simulink library "follow_the_leader_library"  (R2018b)
settings: Solver=VariableStepAuto  StartTime=0.0  StopTime=10.0  RelTol=1e-3
undefined symbols (not defined in the file or in its folder): water, wr
settings Model: Creator=martin  LastModifiedBy=martin

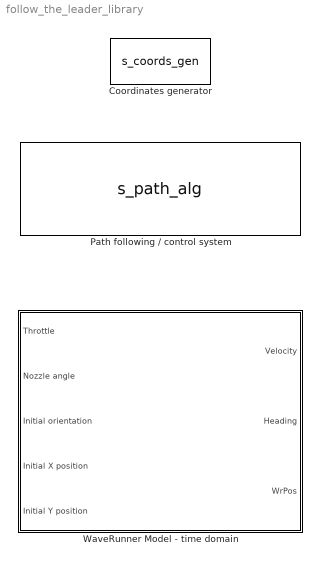
== system follow_the_leader_library ==
  Coordinates generator : S-Function  FunctionName=s_coords_gen  Parameters=steptime fname  SFunctionDeploymentMode=off  EnableBusSupport=off  mask(Coordinates generator){fname=../test1.txt, steptime=1}
      mask prompts: fname "File name"; steptime "Step time [coordinate / sec]"
      mask help:
      | Function simulating a GPS.
      |
      | The file must contain space separated GPS coordinates only, one coordinate / row.
      |
      | The step time controls the rate at which the coordinates are emitted.
      mask Display: fprintf('Coordinates\ngenerator')
  Path following / control system : S-Function  FunctionName=s_path_alg  Parameters=dt g_Kp g_Tf g_Kd g_Ki g_max g_min n_Kp n_Tf n_Kd n_Ki n_max n_min  SFunctionModules='path_alg'  SFunctionDeploymentMode=off  EnableBusSupport=off  mask(Path following / control system){dt=0.5, g_Kp=1.0, g_Tf=1.0, g_Kd=0.0, g_Ki=0.0, g_max=100, g_min=0, n_Kp=-1.0, n_Tf=1.0, n_Kd=0.0, n_Ki=0.0, n_max=6 * pi / 180, n_min=-6 * pi / 180}
      mask prompts: dt "Δt"; g_Kp "Kp"; g_Tf "Tf"; g_Kd "Kd"; g_Ki "Ki"; g_max "Max"; g_min "Min"; n_Kp "Kp"; n_Tf "Tf"; n_Kd "Kd"; n_Ki "Ki"; n_max "Max"; n_min "Min"
      mask DialogControl Container3 Prompt: Controller parameters - Gas
      mask DialogControl Container5 Prompt: Controller parameters - Nozzle angle
      mask Display:
      | text(0.5, 0.5, 'Path Following Algorithm /\nControl system', 'horizontalAlignment', 'center', 'verticalAlignment', 'middle')
      | port_label('input', 1, 'LC coordinates')
      | port_label('input', 2, 'WR position')
      | port_label('input', 3, 'WR angle')
      | port_label('input', 4, 'WR velocity')
      | port_label('output', 1, 'Throttle')
      | port_label('output', 2, 'Nozzle angle')
      | port_label('output', 3, 'Test vector')
  WaveRunner Model - time domain : Subsystem
      mask Display:
      | text(0.5, 0.5, 'WaveRunner model', 'horizontalAlignment', 'center', 'verticalAlignment', 'middle')
      | port_label('input', 1, 'Throttle')
      | port_label('input', 2, 'Nozzle angle')
      | port_label('input', 3, 'Initial orientation')
      | port_label('input', 4, 'Initial X position')
      | port_label('input', 5, 'Initial Y psotion')
      | port_label('output', 1, 'Velocity')
      | port_label('output', 2, 'Heading')
      | port_label('output', 3, 'WaveRunner position')

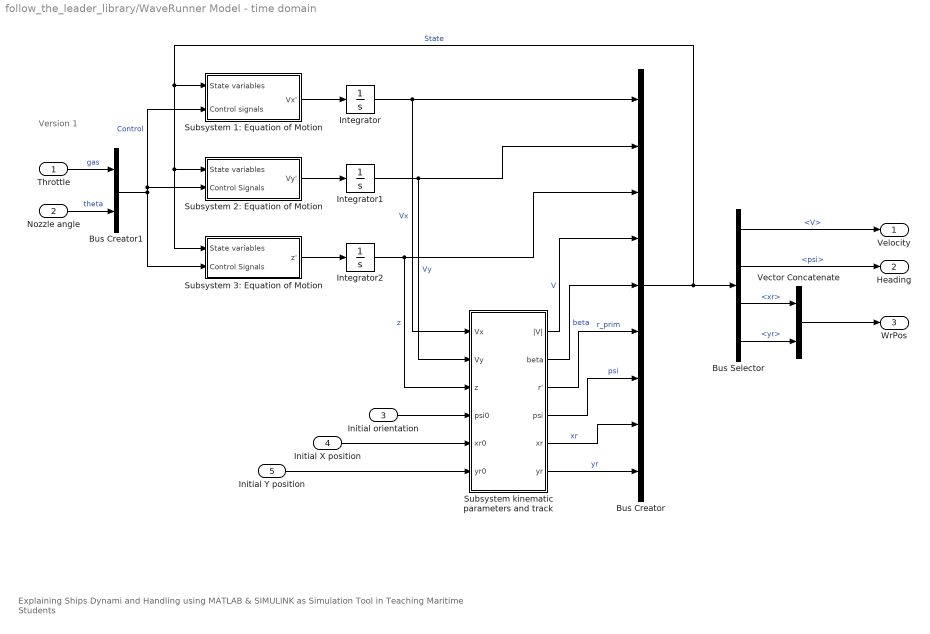
== system follow_the_leader_library/WaveRunner Model - time domain ==
  note: Version 1
  note: Explaining Ships Dynami and Handling using MATLAB & SIMULINK as Simulation Tool in Teaching Maritime Students
  Throttle : Inport
  Nozzle angle : Inport  Port=2
  Initial orientation : Inport  Port=3
  Initial X position : Inport  Port=4
  Initial Y position : Inport  Port=5
  Bus Creator : BusCreator  Inputs=9
  Bus Creator1 : BusCreator  Inputs=2
  Bus Selector : BusSelector  OutputSignals=V,psi,xr,yr
  Integrator : Integrator
  Integrator1 : Integrator
  Integrator2 : Integrator
  Subsystem 1: Equation of Motion : Subsystem
  Subsystem 2: Equation of Motion : Subsystem
  Subsystem 3: Equation of Motion : Subsystem
  Subsystem kinematic parameters and track : Subsystem
  Vector Concatenate : Concatenate
  Velocity : Outport
  Heading : Outport  Port=2
  WrPos : Outport  Port=3
  wires:
  Initial X position/1 -> Subsystem kinematic parameters and track/5(xr0)
  Subsystem 2: Equation of Motion/1(Vy') -> Integrator1/1
  Bus Creator/1 -> Subsystem 3: Equation of Motion/1(State variables), Subsystem 2: Equation of Motion/1(State variables), Subsystem 1: Equation of Motion/1(State variables), Bus Selector/1  "State"
  Integrator2/1 -> Subsystem kinematic parameters and track/3(z), Bus Creator/3  "z"
  Initial orientation/1 -> Subsystem kinematic parameters and track/4(psi0)
  Subsystem kinematic parameters and track/3(r') -> Bus Creator/6  "r_prim"
  Subsystem 1: Equation of Motion/1(Vx') -> Integrator/1
  Subsystem kinematic parameters and track/5(xr) -> Bus Creator/8  "xr"
  Subsystem kinematic parameters and track/6(yr) -> Bus Creator/9  "yr"
  Subsystem kinematic parameters and track/2(beta) -> Bus Creator/5  "beta"
  Bus Creator1/1 -> Subsystem 1: Equation of Motion/2(Control signals), Subsystem 2: Equation of Motion/2(Control Signals), Subsystem 3: Equation of Motion/2(Control Signals)  "Control"
  Subsystem kinematic parameters and track/4(psi) -> Bus Creator/7  "psi"
  Throttle/1 -> Bus Creator1/1  "gas"
  Integrator1/1 -> Subsystem kinematic parameters and track/2(Vy), Bus Creator/2  "Vy"
  Initial Y position/1 -> Subsystem kinematic parameters and track/6(yr0)
  Subsystem 3: Equation of Motion/1(z') -> Integrator2/1
  Subsystem kinematic parameters and track/1(|V|) -> Bus Creator/4  "V"
  Integrator/1 -> Bus Creator/1, Subsystem kinematic parameters and track/1(Vx)  "Vx"
  Bus Selector/2 -> Heading/1  "<psi>"
  Bus Selector/1 -> Velocity/1  "<V>"
  Vector Concatenate/1 -> WrPos/1
  Nozzle angle/1 -> Bus Creator1/2  "theta"
  Bus Selector/3 -> Vector Concatenate/1  "<xr>"
  Bus Selector/4 -> Vector Concatenate/2  "<yr>"

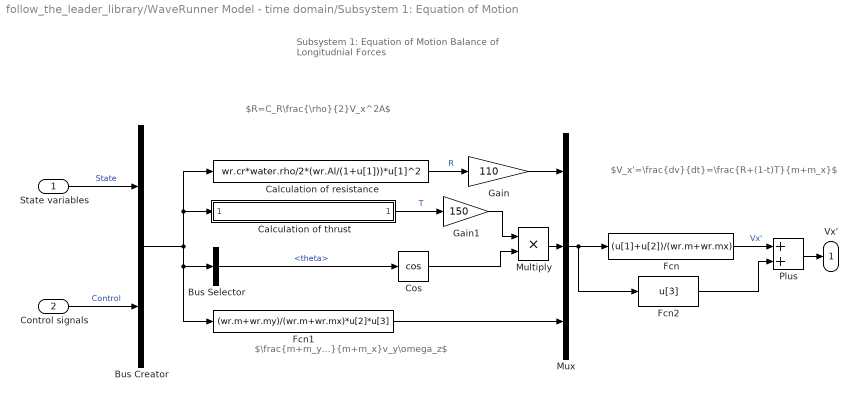
== system follow_the_leader_library/WaveRunner Model - time domain/Subsystem 1: Equation of Motion ==
  note: $\frac{m+m_y}{m+m_x}v_y\omega_z$
  note: Subsystem 1: Equation of Motion
      | Balance of Longitudnial Forces
  note: $V_x'=\frac{dv}{dt}=\frac{R+(1-t)T}{m+m_x}$
  note: $R=C_R\frac{\rho}{2}V_x^2A$
  State variables : Inport
  Control signals : Inport  Port=2
  Bus Creator : BusCreator  Inputs=2  OutDataTypeStr=Bus: slBus1
  Bus Selector : BusSelector  OutputSignals=Control.theta
  Calculation of resistance : Fcn  Expr=wr.cr*water.rho/2*(wr.Al/(1+u[1]))*u[1]^2
  Calculation of thrust : ModelReference  ModelNameDialog=calculation_of_thrust  SimulationMode=Normal  ModelReferenceVersion=1.17
  Cos : Trigonometry  Operator=cos
  Fcn : Fcn  Expr=(u[1]+u[2])/(wr.m+wr.mx)
  Fcn1 : Fcn  Expr=(wr.m+wr.my)/(wr.m+wr.mx)*u[2]*u[3]
  Fcn2 : Fcn  Expr=u[3]
  Gain : Gain  Gain=110
  Gain1 : Gain  Gain=150
  Multiply : Product
  Mux : Mux  Inputs=3
  Plus : Sum
  Vx' : Outport
  wires:
  Mux/1 -> Fcn2/1, Fcn/1
  Calculation of resistance/1 -> Gain/1  "R"
  Control signals/1 -> Bus Creator/2  "Control"
  State variables/1 -> Bus Creator/1  "State"
  Plus/1 -> Vx'/1
  Bus Selector/1 -> Cos/1  "<theta>"
  Fcn1/1 -> Mux/3
  Bus Creator/1 -> Fcn1/1, Bus Selector/1, Calculation of resistance/1, Calculation of thrust/1
  Fcn/1 -> Plus/1  "Vx'"
  Fcn2/1 -> Plus/2
  Multiply/1 -> Mux/2
  Calculation of thrust/1 -> Gain1/1  "T"
  Gain/1 -> Mux/1
  Gain1/1 -> Multiply/1
  Cos/1 -> Multiply/2

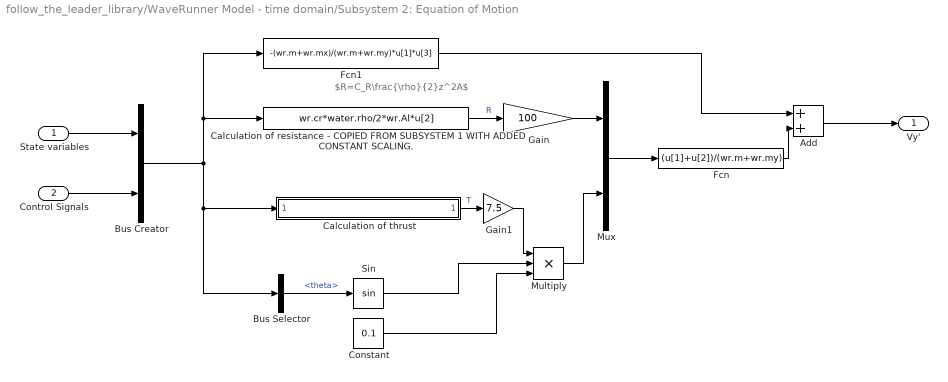
== system follow_the_leader_library/WaveRunner Model - time domain/Subsystem 2: Equation of Motion ==
  note: $R=C_R\frac{\rho}{2}z^2A$
  State variables : Inport
  Control Signals : Inport  Port=2
  Add : Sum
  Bus Creator : BusCreator  Inputs=2
  Bus Selector : BusSelector  OutputSignals=Control.theta
  Calculation of resistance - COPIED FROM SUBSYSTEM 1 WITH ADDED CONSTANT SCALING. : Fcn  Expr=wr.cr*water.rho/2*wr.Al*u[2]
  Calculation of thrust : ModelReference  ModelNameDialog=calculation_of_thrust  SimulationMode=Normal  ModelReferenceVersion=1.17
  Constant : Constant  Value=0.1
  Fcn : Fcn  Expr=(u[1]+u[2])/(wr.m+wr.my)
  Fcn1 : Fcn  Expr=-(wr.m+wr.mx)/(wr.m+wr.my)*u[1]*u[3]
  Gain : Gain  Gain=100
  Gain1 : Gain  Gain=7.5
  Multiply : Product  Inputs=3
  Mux : Mux  Inputs=2
  Sin : Trigonometry
  Vy' : Outport
  wires:
  State variables/1 -> Bus Creator/1
  Control Signals/1 -> Bus Creator/2
  Calculation of resistance - COPIED FROM SUBSYSTEM 1 WITH ADDED CONSTANT SCALING./1 -> Gain/1  "R"
  Sin/1 -> Multiply/2
  Bus Selector/1 -> Sin/1  "<theta>"
  Constant/1 -> Multiply/3
  Bus Creator/1 -> Bus Selector/1, Calculation of thrust/1, Fcn1/1, Calculation of resistance - COPIED FROM SUBSYSTEM 1 WITH ADDED CONSTANT SCALING./1
  Mux/1 -> Fcn/1
  Gain/1 -> Mux/1
  Multiply/1 -> Mux/2
  Fcn/1 -> Add/2
  Fcn1/1 -> Add/1
  Add/1 -> Vy'/1
  Calculation of thrust/1 -> Gain1/1  "T"
  Gain1/1 -> Multiply/1

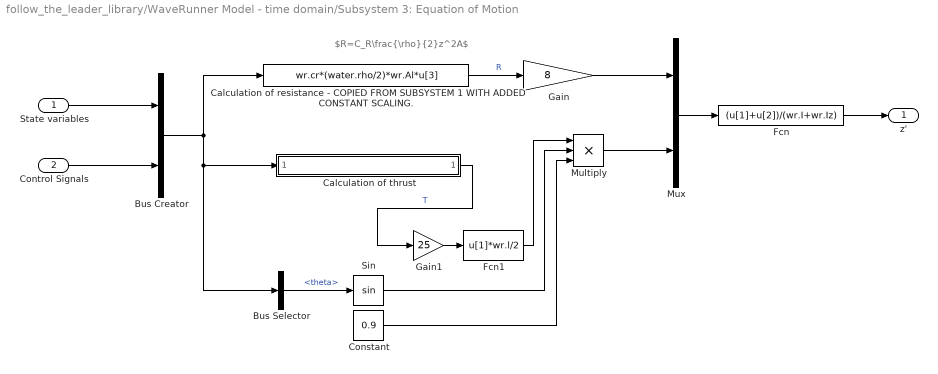
== system follow_the_leader_library/WaveRunner Model - time domain/Subsystem 3: Equation of Motion ==
  note: $R=C_R\frac{\rho}{2}z^2A$
  State variables : Inport
  Control Signals : Inport  Port=2
  Bus Creator : BusCreator  Inputs=2
  Bus Selector : BusSelector  OutputSignals=Control.theta
  Calculation of resistance - COPIED FROM SUBSYSTEM 1 WITH ADDED CONSTANT SCALING. : Fcn  Expr=wr.cr*(water.rho/2)*wr.Al*u[3]
  Calculation of thrust : ModelReference  ModelNameDialog=calculation_of_thrust  SimulationMode=Normal  ModelReferenceVersion=1.17
  Constant : Constant  Value=0.9
  Fcn : Fcn  Expr=(u[1]+u[2])/(wr.I+wr.Iz)
  Fcn1 : Fcn  Expr=u[1]*wr.l/2
  Gain : Gain  Gain=8
  Gain1 : Gain  Gain=25
  Multiply : Product  Inputs=3
  Mux : Mux  Inputs=2
  Sin : Trigonometry
  z' : Outport
  wires:
  Control Signals/1 -> Bus Creator/2
  State variables/1 -> Bus Creator/1
  Sin/1 -> Multiply/2
  Bus Creator/1 -> Calculation of resistance - COPIED FROM SUBSYSTEM 1 WITH ADDED CONSTANT SCALING./1, Bus Selector/1, Calculation of thrust/1
  Calculation of resistance - COPIED FROM SUBSYSTEM 1 WITH ADDED CONSTANT SCALING./1 -> Gain/1  "R"
  Multiply/1 -> Mux/2
  Fcn/1 -> z'/1
  Mux/1 -> Fcn/1
  Gain/1 -> Mux/1
  Fcn1/1 -> Multiply/1
  Constant/1 -> Multiply/3
  Calculation of thrust/1 -> Gain1/1  "T"
  Gain1/1 -> Fcn1/1
  Bus Selector/1 -> Sin/1  "<theta>"

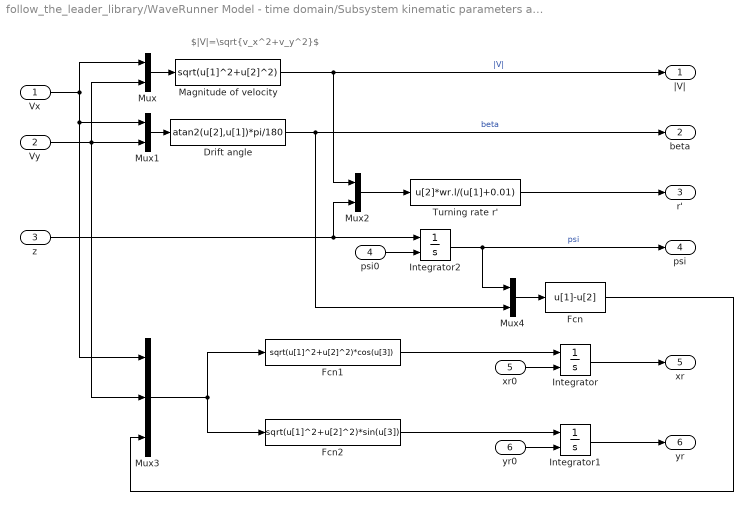
== system follow_the_leader_library/WaveRunner Model - time domain/Subsystem kinematic parameters and track ==
  note: $|V|=\sqrt{v_x^2+v_y^2}$
  Vx : Inport
  Vy : Inport  Port=2
  z : Inport  Port=3
  psi0 : Inport  Port=4
  xr0 : Inport  Port=5
  yr0 : Inport  Port=6
  Drift angle : Fcn  Expr=atan2(u[2],u[1])*pi/180
  Fcn : Fcn  Expr=u[1]-u[2]
  Fcn1 : Fcn  Expr=sqrt(u[1]^2+u[2]^2)*cos(u[3])
  Fcn2 : Fcn  Expr=sqrt(u[1]^2+u[2]^2)*sin(u[3])
  Integrator : Integrator  InitialConditionSource=external
  Integrator1 : Integrator  InitialConditionSource=external
  Integrator2 : Integrator  InitialConditionSource=external
  Magnitude of velocity : Fcn  Expr=sqrt(u[1]^2+u[2]^2)
  Mux{,1..2,4} (4 alike) : Mux  Inputs=2
  Mux3 : Mux  Inputs=3
  Turning rate r' : Fcn  Expr=u[2]*wr.l/(u[1]+0.01)
  |V| : Outport
  beta : Outport  Port=2
  r' : Outport  Port=3
  psi : Outport  Port=4
  xr : Outport  Port=5
  yr : Outport  Port=6
  wires:
  Mux/1 -> Magnitude of velocity/1
  Magnitude of velocity/1 -> Mux2/1, |V|/1  "|V|"
  Vx/1 -> Mux/1, Mux3/1, Mux1/1
  Vy/1 -> Mux/2, Mux3/2, Mux1/2
  Integrator1/1 -> yr/1
  Integrator/1 -> xr/1
  Integrator2/1 -> Mux4/1, psi/1  "psi"
  psi0/1 -> Integrator2/2
  xr0/1 -> Integrator/2
  yr0/1 -> Integrator1/2
  z/1 -> Mux2/2, Integrator2/1
  Mux1/1 -> Drift angle/1
  Drift angle/1 -> Mux4/2, beta/1  "beta"
  Mux2/1 -> Turning rate r'/1
  Turning rate r'/1 -> r'/1
  Mux4/1 -> Fcn/1
  Fcn/1 -> Mux3/3
  Fcn1/1 -> Integrator/1
  Fcn2/1 -> Integrator1/1
  Mux3/1 -> Fcn1/1, Fcn2/1
